simulink model "demo_01"  (R2022a)
settings: Solver=VariableStepAuto  StartTime=0.0  StopTime=50  RelTol=1e-3
libraries: mcbcontrolslib x2, slpidlib x1, simulink x1
settings Model: Creator=ZJH  LastModifiedBy=ZJH

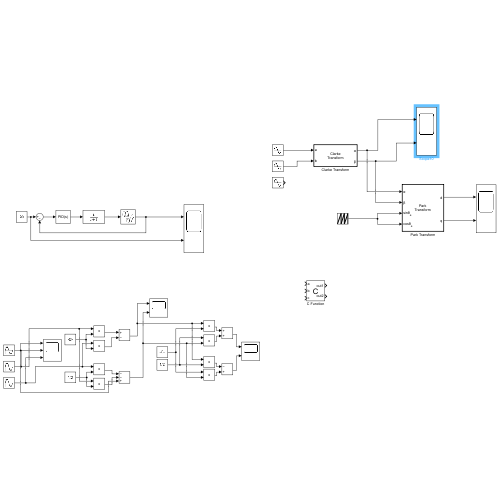
[thumbnail: Simulink's stored preview of the top-level diagram]
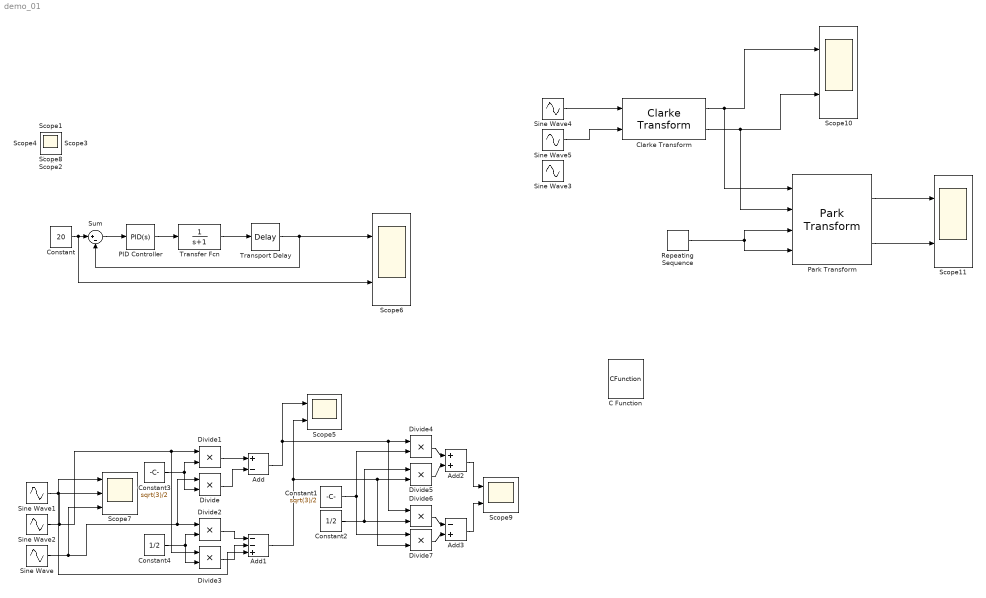
== system demo_01 ==
  Add : Sum  Inputs=+-
  Add1 : Sum  Inputs=--+
  Add2 : Sum
  Add3 : Sum  Inputs=-+
  C Function : CFunction  OutputCode=|
      | out1 = a - (cos(2/3*3.1415926)*b + cos(2/3*3.1415926)*c);
      | out2 =  sin(2/3*3.1415926) ;
  Clarke Transform : mcbcontrolslib/Clarke Transform  VariantControl=Variant2
  Constant : Constant  Value=20
  Constant1 : Constant  Value=sqrt(3)/2
  Constant2 : Constant  Value=1/2
  Constant3 : Constant  Value=sqrt(3)/2
  Constant4 : Constant  Value=1/2
  Divide{,1..7} (8 alike) : Product  Inputs=**
  PID Controller : slpidlib/PID Controller  Controller=PID  Form=Parallel  TimeDomain=Continuous-time  UseExternalTs=off  SampleTime=-1  IntegratorMethod=Forward Euler  FilterMethod=Forward Euler  ControllerParametersSource=internal  P=1.87428300315158  I=2.20630720550221  UseKiTs=off  D=0.115171999854227  N=3.35975749134306  UseFilter=on  TunerSelectOption=Transfer Function Based (PID Tuner App)  InitialConditionSource=internal  InitialConditionForIntegrator=0  InitialConditionForFilter=0  DifferentiatorICPrevScaledInput=0  ExternalReset=none  TrackingMode=off  Kt=1  LimitOutput=off  SatLimitsSource=internal  UpperSaturationLimit=inf  LowerSaturationLimit=-inf  LinearizeAsGain=on  AntiWindupMode=none  Kb=1  POutMin=[]  POutMax=[]  IOutMin=[]  IOutMax=[]  DOutMin=[]  DOutMax=[]  NOutMin=[]  NOutMax=[]  SumOutMin=[]  SumOutMax=[]  SaturationOutMin=[]  SaturationOutMax=[]  PParamMin=[]  PParamMax=[]  IParamMin=[]  IParamMax=[]  DParamMin=[]  DParamMax=[]  NParamMin=[]  NParamMax=[]  KbParamMin=[]  KbParamMax=[]  KtParamMin=[]  KtParamMax=[]  KbOutMin=[]  KbOutMax=[]  KtOutMin=[]  KtOutMax=[]  IntegratorOutMin=[]  IntegratorOutMax=[]  FilterOutMin=[]  FilterOutMax=[]  SumI1OutMin=[]  SumI1OutMax=[]  SumI2OutMin=[]  SumI2OutMax=[]  SumI3OutMin=[]  SumI3OutMax=[]  SumI4OutMin=[]  SumI4OutMax=[]  SumDOutMin=[]  SumDOutMax=[]  DifferentiatorOutMin=[]  DifferentiatorOutMax=[]  FilterDiffOutCoefMin=[]  FilterDiffOutCoefMax=[]  ReciprocalOutMin=[]  ReciprocalOutMax=[]  SumDenOutMin=[]  SumDenOutMax=[]  SumNumOutMin=[]  SumNumOutMax=[]  DivideOutMin=[]  DivideOutMax=[]  UdiffTsProdOutMin=[]  UdiffTsProdOutMax=[]  NTsProdOutMin=[]  NTsProdOutMax=[]  UintegralTsProdOutMin=[]  UintegralTsProdOutMax=[]  UngainTsProdOutMin=[]  UngainTsProdOutMax=[]  IntegratorContinuousStateAttributes=''  IntegratorStateMustResolveToSignalObject=off  IntegratorRTWStateStorageClass=Auto  FilterContinuousStateAttributes=''  FilterStateMustResolveToSignalObject=off  FilterRTWStateStorageClass=Auto  ParallelPVariant=InternalParameters  IdealPVariant=Disabled  IVariant=InternalParameters  DVariant=InternalParameters  IntegratorVariant=Continuous  SatVariant=Disabled  AWVariant=Passthrough  PCopyVariant=Disabled  TRVariant=Disabled  FdbkBlocksVariant=Forward  IdealPFdbkVariant=Disabled  SatFdbkVariant=Disabled  DerivativeFilterVariant=ContFilter  NVariant=InternalParameters  NCopyVariant=Disabled  FilterICVariant=InternalICsFilter  IntegratorICVariant=InternalICs  ExternalResetVariant=Disabled  TRSumVariant=Passthrough  SumFdbkVariant=Disabled  SumVariant=Sum_PID  TsampFilterVariant=InternalTs  TsampNgainVariant=Passthrough  TsampIntegralVariant=Passthrough  ExternalSaturationOutDataTypeStr=Inherit: Same as second input  aMode=0
  Park Transform : mcbcontrolslib/Park Transform  AxisAlignment=D-axis
      settings: SourceProductBaseCode=MT
  Repeating Sequence : simulink/Sources/Repeating Sequence  rep_seq_t=[0 20]  rep_seq_y=[0 360/pi]
  Scope{5..6,9..11} (5 alike) : Scope  NumInputPorts=2
  Scope7 : Scope  NumInputPorts=3
  Sine Wave : Sin  Frequency=0.5  Phase=4/3*pi  SampleTime=0
  Sine Wave1 : Sin  Frequency=0.5  SampleTime=0
  Sine Wave2 : Sin  Frequency=0.5  Phase=2/3*pi  SampleTime=0
  Sine Wave3 : Sin  Frequency=0.5  Phase=4/3*pi  SampleTime=0
  Sine Wave4 : Sin  Frequency=0.5  SampleTime=0
  Sine Wave5 : Sin  Frequency=0.5  Phase=2/3*pi  SampleTime=0
  Sum : Sum  Inputs=|+-
  Transfer Fcn : TransferFcn  Denominator=[1 1]
  Transport Delay : TransportDelay  DelayTime=0.01
  Scope{,1..4,8} (6 alike) : Scope
  wires:
  Sum/1 -> PID Controller/1
  PID Controller/1 -> Transfer Fcn/1
  Transport Delay/1 -> Sum/2, Scope6/1
  Constant/1 -> Scope6/2, Sum/1
  Transfer Fcn/1 -> Transport Delay/1
  Divide1/1 -> Add/1
  Divide/1 -> Add/2
  Sine Wave2/1 -> Scope7/2, Divide3/1, Divide1/1
  Sine Wave/1 -> Scope7/3, Divide/1, Divide2/1
  Sine Wave1/1 -> Add1/3, Scope7/1
  Add/1 -> Divide6/1, Divide4/1, Scope5/1
  Add1/1 -> Divide7/2, Divide5/2, Scope5/2
  Constant3/1 -> Divide/2, Divide1/2
  Constant4/1 -> Divide3/2, Divide2/2
  Divide2/1 -> Add1/1
  Divide3/1 -> Add1/2
  Divide4/1 -> Add2/1
  Divide5/1 -> Add2/2
  Constant1/1 -> Divide7/1, Divide4/2
  Constant2/1 -> Divide6/2, Divide5/1
  Divide6/1 -> Add3/1
  Divide7/1 -> Add3/2
  Add2/1 -> Scope9/1
  Add3/1 -> Scope9/2
  Sine Wave4/1 -> Clarke Transform/1
  Sine Wave5/1 -> Clarke Transform/2
  Clarke Transform/1 -> Park Transform/1, Scope10/1
  Clarke Transform/2 -> Park Transform/2, Scope10/2
  Repeating Sequence/1 -> Park Transform/3, Park Transform/4
  Park Transform/1 -> Scope11/1
  Park Transform/2 -> Scope11/2
